simulink model "test"  (R2018b)
settings: Solver=ode1  StartTime=0.0  StopTime=300000.0  FixedStep=0.1  RelTol=1e-3
settings Model: Creator=user  LastModifiedBy=user

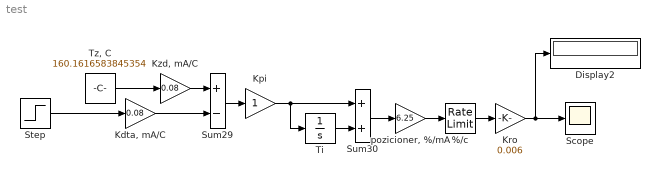
== system test ==
  %/c : RateLimiter  RisingSlewLimit=5  FallingSlewLimit=-5  SampleTimeMode=inherited
  Display2 : Display
  "Kdta, mA/C" : Gain  Gain=0.08
  Kpi : Gain
  Kro : Gain  Gain=0.006
  "Kzd, mA/C" : Gain  Gain=0.08
  Scope : Scope
  Step : Step  After=160  SampleTime=0
  Sum29 : Sum  Inputs=+-
  Sum30 : Sum
  Ti : Integrator  InitialCondition=8000  UpperSaturationLimit=8012  LowerSaturationLimit=6012
  "Tz, C" : Constant  Value=160.1616583845354
  "pozicioner, %/mA" : Gain  Gain=6.25
  wires:
  Step/1 -> "Kdta, mA/C"/1
  "pozicioner, %/mA"/1 -> %/c/1
  "Kzd, mA/C"/1 -> Sum29/1
  "Tz, C"/1 -> "Kzd, mA/C"/1
  Ti/1 -> Sum30/2
  Kro/1 -> Scope/1, Display2/1
  Kpi/1 -> Sum30/1, Ti/1
  "Kdta, mA/C"/1 -> Sum29/2
  %/c/1 -> Kro/1
  Sum30/1 -> "pozicioner, %/mA"/1
  Sum29/1 -> Kpi/1
